simulink model "dc_series_motor_performance_C2000"  (R2024b)
settings: Solver=FixedStepAuto  StartTime=0.0  StopTime=Inf  RelTol=1e-3  EnableMultiTasking=on
values from neighbouring files (symbols this model uses):
  belt_thickness = 0.005    [dc_Series_motor_performance_workspace.mat]
  radius = 0.113    [dc_Series_motor_performance_workspace.mat]
libraries: c2802xlib x3
settings Model: ExtModeTrigDuration=8  Creator=Md Aadil
settings SolverCC: AlgebraicLoopSolver=TrustRegion
settings DataIOCC: ReturnWorkspaceOutputs=off
settings OptimizationCC: DefaultParameterBehavior=Inlined  UseDivisionForNetSlopeComputation=on  UseFloatMulNetSlope=on  DefaultUnderspecifiedDataType=single  InlineInvariantSignals=on  PassReuseOutputArgsAs=Individual arguments  NoFixptDivByZeroProtection=on  EfficientFloat2IntCast=on  LifeSpan=1  MaxStackSize=768  EfficientTunableParamExpr=on
settings DebuggingCC: ParameterTunabilityLossMsg=error  UnconnectedInputMsg=warning  UnconnectedOutputMsg=warning  UnconnectedLineMsg=warning  ArithmeticOperatorsInVariantConditions=warning
settings HardwareCC: ProdBitPerChar=16  ProdBitPerInt=16  ProdBitPerPointer=32  ProdBitPerSizeT=32  ProdBitPerPtrDiffT=32  ProdLargestAtomicInteger=Integer  ProdLargestAtomicFloat=None  ProdWordSize=16  ProdLongLongMode=on  ProdHWDeviceType=Texas Instruments->C2000
settings ModelReferenceCC: EnableRefExpFcnMdlSchedulingChecks=on
settings SFSimCC: SimUseLocalCustomCode=off  MATLABDynamicMemAlloc=off  CustomCodeUndefinedFunction=UseInterfaceOnly
settings RTWCC: Description=Embedded Coder  SystemTargetFile=ert.tlc  HardwareBoard=TI Piccolo F2802x  GenCodeOnly=on  TemplateMakefile=ert_default_tmf  GenerateReport=on  RTWUseLocalCustomCode=off  Toolchain=Texas Instruments Code Composer Studio (C2000)  IncludeHyperlinkInReport=on  LaunchReport=on  CodeProfilingSaveOptions=MetricsOnly  GenerateTraceInfo=on  GenerateTraceReport=on  GenerateTraceReportSl=on  GenerateTraceReportSf=on  GenerateTraceReportEml=on  GenerateCodeMetricsReport=on  GPUComputeCapability=3.5
settings CodeAppCC: ForceParamTrailComments=on  IgnoreCustomStorageClasses=off  OperatorAnnotations=on  SimulinkDataObjDesc=on  SFDataObjDesc=on  MATLABFcnDesc=on  CustomSymbolStrGlobalVar=rt$N$M  CustomSymbolStrType=$N$M  CustomSymbolStrFcn=$N$M$F  CustomSymbolStrMacro=$N$M  InsertBlockDesc=on  StateflowObjectComments=on  MATLABSourceComments=on
settings ERTTargetCC: CodeReplacementLibrary=TI C28x  IncludeMdlTerminateFcn=off  CombineSignalStateStructs=on  SupportComplex=off  SupportContinuousTime=on  SupportNonInlinedSFcns=on  ExtModeTransport=4  ExtModeStaticAlloc=on  ExtModeAutomaticAllocSize=off  ExtModeStaticAllocSize=500  ExtModeMexFile=ext_xcp  ExtModeIntrfLevel=Level2 - Open  ERTFilePackagingFormat=CompactWithDataFile  DynamicArrayContainerType=coder::array

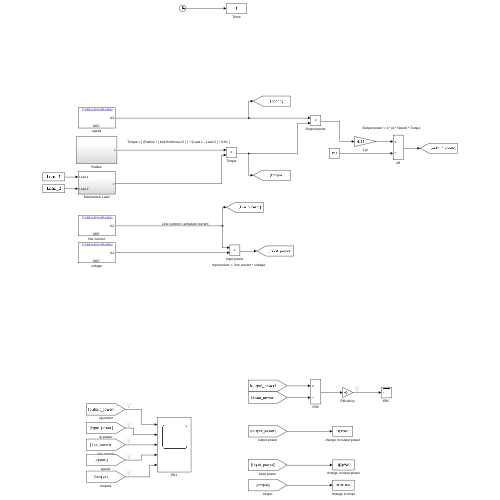
[thumbnail: Simulink's stored preview of the top-level diagram]
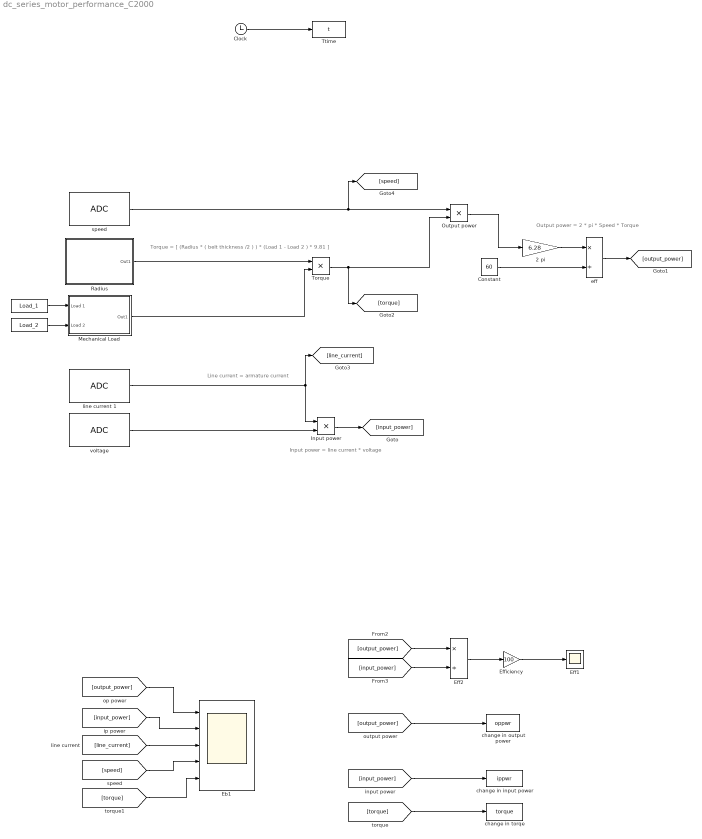
== system dc_series_motor_performance_C2000 ==
  note: Input power = line current * voltage
  note: Line current = armature current
  note: Output power = 2 * pi * Speed * Torque
  note: Torque = [ (Radius * ( belt thickness /2 ) ) * (Load 1 - Load 2 ) * 9.81 ]
  " " : FromWorkspace  VariableName=Load_1  SampleTime=-1
  "  " : FromWorkspace  VariableName=Load_2  SampleTime=-1
  2 pi : Gain  Gain=6.28
  Clock : Clock
  Constant : Constant  Value=60
  Eb1 : Scope  NumInputPorts=5
  "Eff1 " : Scope
  "Eff2 " : Product  Inputs=*/
  "Efficiency " : Gain  Gain=100
  Input power : Product
  Mechanical Load : Subsystem
  Output power : Product
  Radius : Subsystem
  Torque : Product
  Ttime : ToWorkspace  VariableName=t  SampleTime=-1
  "change in input power " : ToWorkspace  VariableName=ippwr  SampleTime=-1
  change in output power : ToWorkspace  VariableName=oppwr  SampleTime=-1
  change in torqe : ToWorkspace  VariableName=torque  SampleTime=-1
  eff : Product  Inputs=*/
  line current 1 : c2802xlib/ADC  blkParamProc=C2000  ADCModule=1  samplingMode=Single sample mode  ADCResolution=12-bit (Single-ended input)  useSOC1=SOC2  useSOC2=SOC0_SOC1  SOCAcquisitionWindow=7  SOCTriggerSource=Software  SOCInterruptTrigger=No ADCINT  Ts=0.001  dType=double  postInterrupt=off  interruptSel=ADCINT1  ADCINTContinuous=on  endma=off  chdma=1  conv1=ADCINA2  conv2=ADCINA0 and ADCINB0  conv1_Type4=ADCIN0  conv2_Type4=ADCIN0 and ADCIN1
  "speed " : c2802xlib/ADC  blkParamProc=C2000  ADCModule=1  samplingMode=Single sample mode  ADCResolution=12-bit (Single-ended input)  useSOC1=SOC3  useSOC2=SOC0_SOC1  SOCAcquisitionWindow=7  SOCTriggerSource=Software  SOCInterruptTrigger=No ADCINT  Ts=0.001  dType=double  postInterrupt=off  interruptSel=ADCINT1  ADCINTContinuous=on  endma=off  chdma=1  conv1=ADCINA3  conv2=ADCINA0 and ADCINB0  conv1_Type4=ADCIN0  conv2_Type4=ADCIN0 and ADCIN1
  voltage : c2802xlib/ADC  blkParamProc=C2000  ADCModule=1  samplingMode=Single sample mode  ADCResolution=12-bit (Single-ended input)  useSOC1=SOC1  useSOC2=SOC0_SOC1  SOCAcquisitionWindow=7  SOCTriggerSource=Software  SOCInterruptTrigger=No ADCINT  Ts=0.001  dType=double  postInterrupt=off  interruptSel=ADCINT1  ADCINTContinuous=on  endma=off  chdma=1  conv1=ADCINA1  conv2=ADCINA0 and ADCINB0  conv1_Type4=ADCIN0  conv2_Type4=ADCIN0 and ADCIN1
  wires:
  [line_current] -> Eb1/3
  [output_power] -> "Eff2 "/1
  [output_power] -> Eb1/1
  [torque] -> change in torqe/1
  [speed] -> Eb1/4
  line current 1/1 -> [line_current], Input power/1
  [output_power] -> change in output power/1
  "speed "/1 -> [speed], Output power/1
  "  "/1 -> Mechanical Load/2(Load 2)
  Torque/1 -> [torque], Output power/2
  [input_power] -> "Eff2 "/2
  voltage/1 -> Input power/2
  Radius/1(Out1) -> Torque/1
  [input_power] -> Eb1/2
  [input_power] -> "change in input power "/1
  Mechanical Load/1(Out1) -> Torque/2
  Clock/1 -> Ttime/1
  Input power/1 -> [input_power]
  " "/1 -> Mechanical Load/1(Load 1)
  [torque] -> Eb1/5
  Constant/1 -> eff/2
  eff/1 -> [output_power]
  2 pi/1 -> eff/1
  Output power/1 -> 2 pi/1
  "Eff2 "/1 -> "Efficiency "/1
  "Efficiency "/1 -> "Eff1 "/1

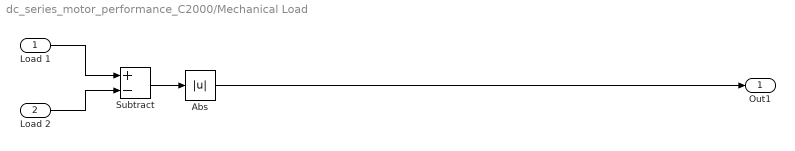
== system dc_series_motor_performance_C2000/Mechanical Load ==
  Load 1 : Inport
  Load 2 : Inport  Port=2
  Abs : Abs  SaturateOnIntegerOverflow=off
  Subtract : Sum  Inputs=+-
  Out1 : Outport
  wires:
  Load 1/1 -> Subtract/1
  Load 2/1 -> Subtract/2
  Abs/1 -> Out1/1
  Subtract/1 -> Abs/1

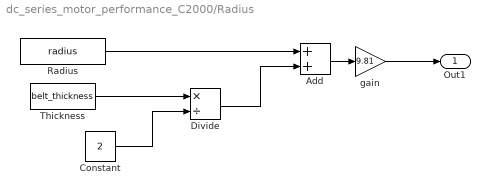
== system dc_series_motor_performance_C2000/Radius ==
  Add : Sum
  Constant : Constant  Value=2
  Divide : Product  Inputs=*/
  Radius : Constant  Value=radius  SampleTime=-1
  Thickness : Constant  Value=belt_thickness  SampleTime=-1
  gain : Gain  Gain=9.81
  Out1 : Outport
  wires:
  Radius/1 -> Add/1
  Add/1 -> gain/1
  gain/1 -> Out1/1
  Thickness/1 -> Divide/1
  Divide/1 -> Add/2
  Constant/1 -> Divide/2
